simulink model "dstatcom_avg"  (Simulink 7.9)
settings: Solver=ode23tb  SolverMode=SingleTasking  StartTime=0.0  StopTime=12  FixedStep=Ts  MaxStep=1/60  RelTol=1e-4
InitFcn:
  | Ts=40e-6;
  | tic;
StopFcn:
  | toc;
undefined symbols (not defined in the file or in its folder): D11, Delta, DiscIntNeverNeededParam
libraries: powerlib x53, powerlib_extras x39
(part 1 of 2)
Description:
  | Copyright 2008-2012 The MathWorks, Inc.
settings Model: Creator=MathWorks  LastModifiedBy=ywlaw  ExtModeTrigMode=oneshot  ExtModeArmWhenConnect=off  ExtModeAutoUpdateStatusClock=off
settings DataIOCC: LimitDataPoints=off  SaveFinalState=on  SaveFormat=Structure  SaveOutput=off  SaveTime=off  SignalLoggingName=sigsOut
settings OptimizationCC: BlockReduction=off  BooleanDataType=off  InitFltsAndDblsToZero=on
settings DebuggingCC: SaveWithParameterizedLinksMsg=none  SignalResolutionControl=TryResolveAllWithWarning  SolverPrmCheckMsg=none  MultiTaskDSMMsg=warning  MultiTaskCondExecSysMsg=none  FcnCallInpInsideContextMsg=Use local settings  StrictBusMsg=None
settings HardwareCC: TargetUnknown=on
settings RTWCC: IncludeERTFirstTime=on
settings GRTTargetCC: TargetFcnLib=ansi_tfl_tmw.mat  CombineOutputUpdateFcns=off  GRTInterface=on

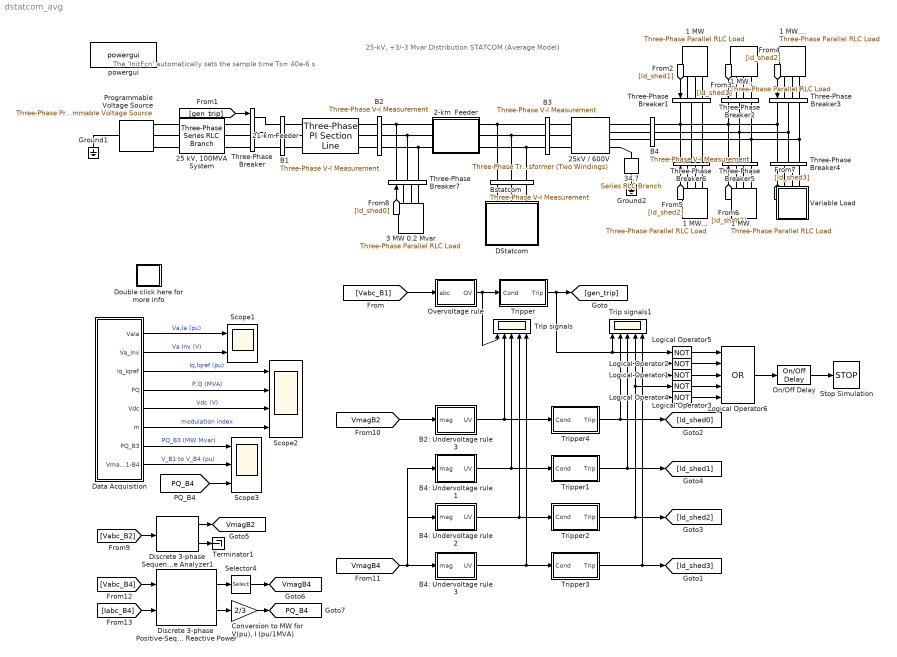
== system dstatcom_avg ==
  note: 25-kV, +3/-3 Mvar Distribution STATCOM (Average Model)
  note: The 'InitFcn' automatically sets
      |  the sample time Ts= 40e-6 s
  1 MW : powerlib/Elements/Three-Phase Parallel RLC Load  LConnTagsString=A|B|C  Configuration=Y (floating)  NominalVoltage=600  NominalFrequency=60  ActivePower=1e6  InductivePower=0  CapacitivePower=0  Measurements=None  LoadType=constant Z
  1 MW. : powerlib/Elements/Three-Phase Parallel RLC Load  LConnTagsString=A|B|C  Configuration=Y (floating)  NominalVoltage=600  NominalFrequency=60  ActivePower=1e6  InductivePower=0  CapacitivePower=0  Measurements=None  LoadType=constant Z
  1 MW.. : powerlib/Elements/Three-Phase Parallel RLC Load  LConnTagsString=A|B|C  Configuration=Y (floating)  NominalVoltage=600  NominalFrequency=60  ActivePower=1e6  InductivePower=0  CapacitivePower=0  Measurements=None  LoadType=constant Z
  1 MW... : powerlib/Elements/Three-Phase Parallel RLC Load  LConnTagsString=A|B|C  Configuration=Y (floating)  NominalVoltage=600  NominalFrequency=60  ActivePower=1e6  InductivePower=0  CapacitivePower=0  Measurements=None  LoadType=constant Z
  1 MW.... : powerlib/Elements/Three-Phase Parallel RLC Load  LConnTagsString=A|B|C  Configuration=Y (floating)  NominalVoltage=600  NominalFrequency=60  ActivePower=1e6  InductivePower=0  CapacitivePower=0  Measurements=None  LoadType=constant Z
  2-km  Feeder : Subsystem
      mask Display: plot(0,0,100,100,[20,20,80,80,90,80,80,20,20,10],[50,40,40,50,50,50,61,61,50,50])
  21-km Feeder : powerlib/Elements/Three-Phase PI Section Line  LConnTagsString=a|b|c  RConnTagsString=A|B|C  Frequency=60  Resistances=[0.1153 0.3963]  Inductances=[1.048e-3 2.730e-3]  Capacitances=[11.33e-9 5.338e-9]  Length=21
  "25 kV, 100MVA System" : powerlib/Elements/Three-Phase Series RLC Branch  LConnTagsString=A|B|C  RConnTagsString=A|B|C  BranchType=RL  Resistance=25e3^2/100e6/10  Inductance=25e3^2/100e6/(2*pi*60)  Capacitance=1.0  Measurements=None
  25kV / 600V : powerlib/Elements/Three-Phase Transformer (Two Windings)  Winding1Connection=Delta (D11)  UNITS=pu  NominalPower=[6e6 60]  Winding1=[25e3 , 0.05/30/2 , 0.05]  Winding2Connection=Yn  Winding2=[600 , 0.05/30/2 , 0]  SetSaturation=off  Rm=500  Lm=500  Saturation="[ 0,0  ;  0.005,1.2  ;  1.0,1.4 ]"  Hysteresis=off  DataFile='basic_model'  SetInitialFlux=off  InitialFluxes=[ 0.8 , -0.8 , 0.7 ]  Measurements=None  MoreParameters=off  BreakLoop=off  DataType=off  TransfoNumber=1
  3 MW 0.2 Mvar : powerlib/Elements/Three-Phase Parallel RLC Load  LConnTagsString=A|B|C  Configuration=Y (grounded)  NominalVoltage=25e3  NominalFrequency=60  ActivePower=3e6  InductivePower=0  CapacitivePower=0.2e6  Measurements=None  LoadType=constant Z
  34.7 : powerlib/Elements/Series RLC Branch  LConnTagsString=__new0  RConnTagsString=__new0  BranchType=R  Resistance=34.7  Inductance=1.0  SetiL0=off  InitialCurrent=0  Capacitance=1.0  Setx0=off  InitialVoltage=0  Measurements=None
  B1 : powerlib/Measurements/Three-Phase V-I Measurement  VoltageMeasurement=phase-to-ground  SetLabelV=on  LabelV=Vabc_B1  Vpu=on  VpuLL=off  CurrentMeasurement=no  SetLabelI=off  LabelI=Iabc  Ipu=off  Pbase=100e6  Vbase=25e3  OutputType=Complex  PhasorSimulation=off  PSBequivalent=0
  B2 : powerlib/Measurements/Three-Phase V-I Measurement  VoltageMeasurement=phase-to-ground  SetLabelV=on  LabelV=Vabc_B2  Vpu=on  VpuLL=off  CurrentMeasurement=no  SetLabelI=off  LabelI=Iabc  Ipu=off  Pbase=100e6  Vbase=25e3  OutputType=Complex  PhasorSimulation=off  PSBequivalent=0
  B2: Undervoltage rule 3 : Subsystem  mask{Freq=60, Vmin=[ 0.94, 6 ]}
      mask prompts: Freq "Fundamental frequency (Hz)"; Vmin "[Minimum voltage (p.u.), Delay (s)]"
      mask init:
      | Min_V1 = Vmin(1);
      | Delay_V1 = Vmin(2);
      | a = exp(2*pi*j/3);
      | a2 = a^2;
  B3 : powerlib/Measurements/Three-Phase V-I Measurement  VoltageMeasurement=phase-to-ground  SetLabelV=on  LabelV=Vabc_B3  Vpu=on  VpuLL=off  CurrentMeasurement=yes  SetLabelI=on  LabelI=Iabc_B3  Ipu=on  Pbase=1e6  Vbase=25e3  OutputType=Magnitude  PhasorSimulation=off  PSBequivalent=0
  B4 : powerlib/Measurements/Three-Phase V-I Measurement  VoltageMeasurement=phase-to-ground  SetLabelV=on  LabelV=Vabc_B4  Vpu=on  VpuLL=off  CurrentMeasurement=yes  SetLabelI=on  LabelI=Iabc_B4  Ipu=on  Pbase=1e6  Vbase=600  OutputType=Magnitude  PhasorSimulation=off  PSBequivalent=0
  B4: Undervoltage rule 1 : Subsystem  mask{Freq=60, Vmin=[ 0.94, 6 ]}
      mask prompts: Freq "Fundamental frequency (Hz)"; Vmin "[Minimum voltage (p.u.), Delay (s)]"
      mask init:
      | Min_V1 = Vmin(1);
      | Delay_V1 = Vmin(2);
      | a = exp(2*pi*j/3);
      | a2 = a^2;
  B4: Undervoltage rule 2 : Subsystem  mask{Freq=60, Vmin=[ 0.92, 3 ]}
      mask prompts: Freq "Fundamental frequency (Hz)"; Vmin "[Minimum voltage (p.u.), Delay (s)]"
      mask init:
      | Min_V1 = Vmin(1);
      | Delay_V1 = Vmin(2);
      | a = exp(2*pi*j/3);
      | a2 = a^2;
  B4: Undervoltage rule 3 : Subsystem  mask{Freq=60, Vmin=[ 0.90, 1.5 ]}
      mask prompts: Freq "Fundamental frequency (Hz)"; Vmin "[Minimum voltage (p.u.), Delay (s)]"
      mask init:
      | Min_V1 = Vmin(1);
      | Delay_V1 = Vmin(2);
      | a = exp(2*pi*j/3);
      | a2 = a^2;
  Bstatcom : powerlib/Measurements/Three-Phase V-I Measurement  VoltageMeasurement=phase-to-ground  SetLabelV=on  LabelV=Vabc_Bstatcom  Vpu=on  VpuLL=off  CurrentMeasurement=yes  SetLabelI=on  LabelI=Iabc_Bstatcom  Ipu=on  Pbase=3e6  Vbase=25e3  OutputType=Magnitude  PhasorSimulation=off  PSBequivalent=0
  "Conversion to MW for V(pu), I (pu/1MVA)" : Gain  Gain=2/3  SaturateOnIntegerOverflow=on  OutDataTypeStr=Inherit: Same as input  ParamDataTypeStr=Inherit: Same as input
  DStatcom : Subsystem
      mask Display: disp('D-STATCOM\n+/- 3Mvar\nAverage')
  Data Acquisition : Subsystem
  Discrete 3-phase Sequence Analyzer1 : powerlib_extras/Discrete Measurements/Discrete 3-phase Sequence Analyzer  Freq=60  n=1  seq=Positive  Par_Init=[1 0]  Ts=Ts
  Discrete 3-phase  Positive-Sequence  Active & Reactive Power : powerlib_extras/Discrete Measurements/Discrete 3-phase  Positive-Sequence  Active & Reactive Power  Freq=60  Par_Vinit=[1 0]  Par_Iinit=[0 0]  Ts=Ts
  Double click here for more info : Subsystem
      settings: OpenFcn=showdemo(bdroot(gcb))
      mask Display: disp('?')
  Ground1 : powerlib/Elements/Ground  LConnTagsString=a
  Ground2 : powerlib/Elements/Ground  LConnTagsString=a
  Logical Operator{1..5} (5 alike) : Logic  Operator=NOT  AllPortsSameDT=off
  Logical Operator6 : Logic  Operator=OR  Inputs=5  AllPortsSameDT=off
  On/Off Delay : powerlib_extras/Control  Blocks/On//Off Delay  type_delay=On delay  delay=0.1  ic=0
  Overvoltage rule : Subsystem  mask{Freq=60, Vmax=[ 1.1, 1.5 ]}
      mask prompts: Freq "Fundamental frequency (Hz)"; Vmax "[Maximum voltage (p.u.), Delay (s)]"
      mask init:
      | Max_V1 = Vmax(1);
      | Delay_V1 = Vmax(2);
      | a = exp(2*pi*j/3);
      | a2 = a^2;
  Programmable Voltage Source : powerlib/Electrical Sources/Three-Phase Programmable Voltage Source  PositiveSequence=[(26925)*1 0 60]  VariationEntity=None  VariationType=Table of time-amplitude pairs  VariationTypeAlt=Step  VariationStep=0.5  VariationRate=10  VariationMagnitude=0.3  VariationFrequency=2  VariationTiming=[1 2]  VariationPhaseA=off  Amplitudes=[1 1.06 0.94 1.0]  TimeValues=[0 0.2 0.3 0.4]  HarmonicGeneration=off  HarmonicA=[3 0.2 -25 0]  HarmonicB=[2 0.15 35 2]  Timing="[0.05  3]"  BusType=swing  Pref=0  Qref=0  Qmin=-inf  Qmax=inf
  Scope1 : Scope  NumInputPorts=2
      settings: TimeRange=0.5  YMin=-1.5~-4000  YMax=1.5~4000  SaveName=Sig1  SampleInput=on  SampleTime=Ts
  Scope2 : Scope  NumInputPorts=4
      settings: ShowLegends=on  TimeRange=1  YMin=-1.5~-4~2200~0.4  YMax=1.5~4~2600~1.2  SaveName=Scope2  SampleInput=on  SampleTime=Ts*32
  Scope3 : Scope  NumInputPorts=3
      settings: ShowLegends=on  TimeRange=1  YMin=0~0.725~-3.5  YMax=6~1~3.5  SaveName=Scope3  SampleInput=on  SampleTime=Ts
  Selector4 : Selector  InputPortWidth=2  IndexOptions=Index vector (dialog)  Indices=1  OutputSizes=1
  Stop Simulation : Stop
  Terminator1 : Terminator
  Three-Phase Breaker{,1..7} (8 alike) : powerlib/Elements/Three-Phase Breaker  InitialState=closed  SwitchA=on  SwitchB=on  SwitchC=on  SwitchTimes="[4/60  10/60]"  External=on  BreakerResistance=0.001  SnubberResistance=1e6  SnubberCapacitance=inf  Measurements=None
  Trip signals : Scope  NumInputPorts=5
      settings: ShowLegends=on  YMin=0~-5~-5~-5~-5  YMax=6~5~5~5~5  SaveName=Sig10  SampleInput=on  SampleTime=Ts
  Trip signals1 : Scope  NumInputPorts=5
      settings: ShowLegends=on  TimeRange=0.5  YMin=0~-5~-5~-5~-5  YMax=6~5~5~5~5  SaveName=Sig11  SampleInput=on  SampleTime=Ts
  Tripper : Subsystem
  Tripper1 : Subsystem
  Tripper2 : Subsystem
  Tripper3 : Subsystem
  Tripper4 : Subsystem
  Variable Load : Subsystem  mask(Variable Load (Constant Current)){Par_Nom=[3000 0.9], Par_Mod=[2000  5], Par_Time=[0.15 20], Vbase=600, Ts=Ts}
      mask prompts: Par_Nom "Nominal load: [ Current (Arms)    Power factor (0 a 1) ]"; Par_Mod "Modulation: [ Amplitude (Arms)   Frequency (Hz) ]"; Par_Time "Modulation timing : [ Ton  Toff ]"; Vbase "Nominal voltage (Volts rms ph-ph)"; Ts "Sample time:"
      mask init:
      | NomAmp=Par_Nom(1)*sqrt(2);
      | NomPha=-acos(Par_Nom(2));
      | ModFreq=Par_Mod(2);
      | ModAmp=Par_Mod(1)*sqrt(2);
      | Ton=Par_Time(1);
      | Toff=Par_Time(2);
  powergui : powerlib/powergui  Priority=2  SimulationMode=Discrete  SolverType=Tustin  SampleTime=Ts  frequency=60  SPID=off  DisableSnubberDevices=off  DisableRonSwitches=off  DisableVfSwitches=off  SwTol=0  Interpol=off  DisplayEquations=off  FunctionMessages=off  frequencyindice=0  Pbase=100e6  ErrMax=1e-4  Iterations=50  UnitsV=kV  UnitsW=MW  echomessages=off  HookPort=off  EnableUseOfTLC=off  x0status=blocks  RestoreLinks=warning  ResistiveCurrentMeasurement=off  Frange=[0:2:500]  Ylog=off  Xlog=on  ShowGrid=off  save=off  variable=ZData  structure=Sig1  ZoomFFT=on  StartTime=0.26  cycles=2  DisplayStyle=1  fundamental=60  FreqAxis=off  MaxFrequency=5000  frequencyindicesteady=1  RmsSteady=1  display=off  Ts=0  methode=off
  tag scope: PQ_B4=global, VmagB2=global, VmagB4=global
  wires:
  Data Acquisition/1(VaIa) -> Scope1/1  "Va,Ia (pu)"
  Data Acquisition/2(Va_Inv) -> Scope1/2  "Va Inv (V)"
  Data Acquisition/5(Vdc) -> Scope2/3  "Vdc (V)"
  Data Acquisition/4(PQ) -> Scope2/2  "P,Q (MVA)"
  Data Acquisition/3(Iq_Iqref) -> Scope2/1  "Iq,Iqref (pu)"
  Data Acquisition/6(m) -> Scope2/4  "modulation index"
  Data Acquisition/7(PQ_B3) -> Scope3/1  "PQ_B3 (MW Mvar)"
  Data Acquisition/8(VmagB1-B4) -> Scope3/2  "V_B1 to V_B4 (pu)"
  [gen_trip] -> Three-Phase Breaker/1
  [ld_shed1] -> Three-Phase Breaker1/1
  [ld_shed1] -> Three-Phase Breaker2/1
  [ld_shed2] -> Three-Phase Breaker3/1
  [ld_shed2] -> Three-Phase Breaker6/1
  [ld_shed3] -> Three-Phase Breaker5/1
  [ld_shed3] -> Three-Phase Breaker4/1
  Overvoltage rule/1(OV) -> Tripper/1(Cond), Trip signals/1
  Tripper/1(Trip) -> [gen_trip], Trip signals1/1, Logical Operator5/1
  Tripper1/1(Trip) -> [ld_shed1], Trip signals1/3, Logical Operator1/1
  Tripper2/1(Trip) -> [ld_shed2], Trip signals1/4, Logical Operator3/1
  Tripper3/1(Trip) -> [ld_shed3], Trip signals1/5, Logical Operator4/1
  [Vabc_B1] -> Overvoltage rule/1(abc)
  [VmagB4] -> B4: Undervoltage rule 1/1(mag), B4: Undervoltage rule 2/1(mag), B4: Undervoltage rule 3/1(mag)
  B4: Undervoltage rule 1/1(UV) -> Tripper1/1(Cond), Trip signals/3
  B4: Undervoltage rule 2/1(UV) -> Tripper2/1(Cond), Trip signals/4
  B4: Undervoltage rule 3/1(UV) -> Tripper3/1(Cond), Trip signals/5
  [ld_shed0] -> Three-Phase Breaker7/1
  Tripper4/1(Trip) -> [ld_shed0], Trip signals1/2, Logical Operator2/1
  B2: Undervoltage rule 3/1(UV) -> Tripper4/1(Cond), Trip signals/2
  [Vabc_B2] -> Discrete 3-phase Sequence Analyzer1/1
  Discrete 3-phase Sequence Analyzer1/2 -> Terminator1/1
  Discrete 3-phase Sequence Analyzer1/1 -> [VmagB2]
  [VmagB2] -> B2: Undervoltage rule 3/1(mag)
  [Vabc_B4] -> Discrete 3-phase  Positive-Sequence  Active & Reactive Power/1
  [Iabc_B4] -> Discrete 3-phase  Positive-Sequence  Active & Reactive Power/2
  Discrete 3-phase  Positive-Sequence  Active & Reactive Power/2 -> "Conversion to MW for V(pu), I (pu/1MVA)"/1
  Discrete 3-phase  Positive-Sequence  Active & Reactive Power/1 -> Selector4/1
  Selector4/1 -> [VmagB4]
  "Conversion to MW for V(pu), I (pu/1MVA)"/1 -> [PQ_B4]
  [PQ_B4] -> Scope3/3
  Logical Operator5/1 -> Logical Operator6/1
  Logical Operator2/1 -> Logical Operator6/2
  Logical Operator1/1 -> Logical Operator6/3
  Logical Operator3/1 -> Logical Operator6/4
  Logical Operator4/1 -> Logical Operator6/5
  Logical Operator6/1 -> On/Off Delay/1
  On/Off Delay/1 -> Stop Simulation/1
  connections:
  B3/LConn2 -- 2-km  Feeder/RConn2 -- Bstatcom/LConn2
  2-km  Feeder/RConn1 -- B3/LConn1 -- Bstatcom/LConn1
  B3/LConn3 -- 2-km  Feeder/RConn3 -- Bstatcom/LConn3
  34.7/RConn1 -- Ground2/LConn1
  25kV / 600V/RConn4 -- 34.7/LConn1
  Programmable Voltage Source/RConn1 -- "25 kV, 100MVA System"/LConn1
  Programmable Voltage Source/RConn2 -- "25 kV, 100MVA System"/LConn2
  Programmable Voltage Source/RConn3 -- "25 kV, 100MVA System"/LConn3
  Ground1/LConn1 -- Programmable Voltage Source/LConn1
  21-km Feeder/RConn1 -- B2/LConn1
  21-km Feeder/RConn2 -- B2/LConn2
  21-km Feeder/RConn3 -- B2/LConn3
  2-km  Feeder/LConn1 -- B2/RConn1 -- Three-Phase Breaker7/RConn1
  2-km  Feeder/LConn2 -- B2/RConn2 -- Three-Phase Breaker7/RConn2
  Bstatcom/RConn3 -- DStatcom/RConn3
  DStatcom/RConn1 -- Bstatcom/RConn1
  DStatcom/RConn2 -- Bstatcom/RConn2
  B3/RConn1 -- 25kV / 600V/LConn1
  B3/RConn2 -- 25kV / 600V/LConn2
  B3/RConn3 -- 25kV / 600V/LConn3
  25kV / 600V/RConn1 -- B4/RConn1
  25kV / 600V/RConn2 -- B4/RConn2
  25kV / 600V/RConn3 -- B4/RConn3
  Three-Phase Breaker3/RConn1 -- Three-Phase Breaker2/RConn1 -- Three-Phase Breaker1/RConn1 -- B4/LConn1 -- Three-Phase Breaker6/RConn1 -- Three-Phase Breaker5/RConn1 -- Three-Phase Breaker4/RConn1
  Three-Phase Breaker2/RConn3 -- B4/LConn3 -- Three-Phase Breaker1/RConn3 -- Three-Phase Breaker6/RConn3 -- Three-Phase Breaker5/RConn3 -- Three-Phase Breaker3/RConn3 -- Three-Phase Breaker4/RConn3
  "25 kV, 100MVA System"/RConn1 -- Three-Phase Breaker/LConn1
  "25 kV, 100MVA System"/RConn2 -- Three-Phase Breaker/LConn2
  "25 kV, 100MVA System"/RConn3 -- Three-Phase Breaker/LConn3
  Three-Phase Breaker/RConn2 -- B1/LConn2
  Three-Phase Breaker/RConn3 -- B1/LConn3
  Three-Phase Breaker/RConn1 -- B1/LConn1
  2-km  Feeder/LConn3 -- B2/RConn3 -- Three-Phase Breaker7/RConn3
  B1/RConn1 -- 21-km Feeder/LConn1
  B1/RConn2 -- 21-km Feeder/LConn2
  B1/RConn3 -- 21-km Feeder/LConn3
  Three-Phase Breaker1/LConn3 -- 1 MW/LConn3
  Three-Phase Breaker1/LConn2 -- 1 MW/LConn2
  Three-Phase Breaker1/LConn1 -- 1 MW/LConn1
  Three-Phase Breaker2/LConn3 -- 1 MW../LConn3
  Three-Phase Breaker2/LConn2 -- 1 MW../LConn2
  Three-Phase Breaker2/LConn1 -- 1 MW../LConn1
  1 MW..../LConn1 -- Three-Phase Breaker3/LConn1
  1 MW..../LConn2 -- Three-Phase Breaker3/LConn2
  1 MW..../LConn3 -- Three-Phase Breaker3/LConn3
  Variable Load/LConn1 -- Three-Phase Breaker4/LConn1
  Variable Load/LConn2 -- Three-Phase Breaker4/LConn2
  Variable Load/LConn3 -- Three-Phase Breaker4/LConn3
  1 MW./LConn1 -- Three-Phase Breaker5/LConn1
  1 MW./LConn2 -- Three-Phase Breaker5/LConn2
  1 MW./LConn3 -- Three-Phase Breaker5/LConn3
  Three-Phase Breaker2/RConn2 -- B4/LConn2 -- Three-Phase Breaker1/RConn2 -- Three-Phase Breaker6/RConn2 -- Three-Phase Breaker5/RConn2 -- Three-Phase Breaker3/RConn2 -- Three-Phase Breaker4/RConn2
  1 MW.../LConn1 -- Three-Phase Breaker6/LConn1
  1 MW.../LConn2 -- Three-Phase Breaker6/LConn2
  1 MW.../LConn3 -- Three-Phase Breaker6/LConn3
  Three-Phase Breaker7/LConn1 -- 3 MW 0.2 Mvar/LConn1
  Three-Phase Breaker7/LConn2 -- 3 MW 0.2 Mvar/LConn2
  Three-Phase Breaker7/LConn3 -- 3 MW 0.2 Mvar/LConn3

== system dstatcom_avg/2-km  Feeder ==
  Three-Phase Mutual Inductance Z1-Z0 : powerlib/Elements/Three-Phase Mutual Inductance Z1-Z0  LConnTagsString=a|b|c  RConnTagsString=A|B|C  PositiveSequence="[0.1153  1.048e-3]*2"  ZeroSequence="[0.3963  2.730e-3]*2"
  A : PMIOPort  Port=1  Side=Left
  B : PMIOPort  Port=2  Side=Left
  "C " : PMIOPort  Port=3  Side=Left
  a : PMIOPort  Port=4  Side=Right
  b : PMIOPort  Port=5  Side=Right
  c : PMIOPort  Port=6  Side=Right
  connections:
  Three-Phase Mutual Inductance Z1-Z0/RConn3 -- c/RConn1
  Three-Phase Mutual Inductance Z1-Z0/RConn2 -- b/RConn1
  Three-Phase Mutual Inductance Z1-Z0/RConn1 -- a/RConn1
  "C "/RConn1 -- Three-Phase Mutual Inductance Z1-Z0/LConn3
  B/RConn1 -- Three-Phase Mutual Inductance Z1-Z0/LConn2
  A/RConn1 -- Three-Phase Mutual Inductance Z1-Z0/LConn1

== system dstatcom_avg/B2: Undervoltage rule 3 ==
  mag : Inport
  On/Off Delay : powerlib_extras/Control  Blocks/On//Off Delay  type_delay=On delay  delay=Delay_V1  ic=0
  Relational Operator : RelationalOperator  Operator=<  OutDataTypeStr=boolean
  V0/V1 max1 : Constant  Value=Min_V1
  UV : Outport
  wires:
  V0/V1 max1/1 -> Relational Operator/2
  mag/1 -> Relational Operator/1
  Relational Operator/1 -> On/Off Delay/1
  On/Off Delay/1 -> UV/1

== system dstatcom_avg/B4: Undervoltage rule 1 ==
  mag : Inport
  On/Off Delay : powerlib_extras/Control  Blocks/On//Off Delay  type_delay=On delay  delay=Delay_V1  ic=0
  Relational Operator : RelationalOperator  Operator=<  OutDataTypeStr=boolean
  V0/V1 max1 : Constant  Value=Min_V1
  UV : Outport
  wires:
  V0/V1 max1/1 -> Relational Operator/2
  mag/1 -> Relational Operator/1
  Relational Operator/1 -> On/Off Delay/1
  On/Off Delay/1 -> UV/1

== system dstatcom_avg/B4: Undervoltage rule 2 ==
  mag : Inport
  On/Off Delay2 : powerlib_extras/Control  Blocks/On//Off Delay  type_delay=On delay  delay=Delay_V1  ic=0
  Relational Operator7 : RelationalOperator  Operator=<
  V0/V1 max5 : Constant  Value=Min_V1
  UV : Outport
  wires:
  On/Off Delay2/1 -> UV/1
  V0/V1 max5/1 -> Relational Operator7/2
  mag/1 -> Relational Operator7/1
  Relational Operator7/1 -> On/Off Delay2/1

== system dstatcom_avg/B4: Undervoltage rule 3 ==
  mag : Inport
  On/Off Delay2 : powerlib_extras/Control  Blocks/On//Off Delay  type_delay=On delay  delay=Delay_V1  ic=0
  Relational Operator7 : RelationalOperator  Operator=<
  V0/V1 max5 : Constant  Value=Min_V1
  UV : Outport
  wires:
  On/Off Delay2/1 -> UV/1
  V0/V1 max5/1 -> Relational Operator7/2
  Relational Operator7/1 -> On/Off Delay2/1
  mag/1 -> Relational Operator7/1

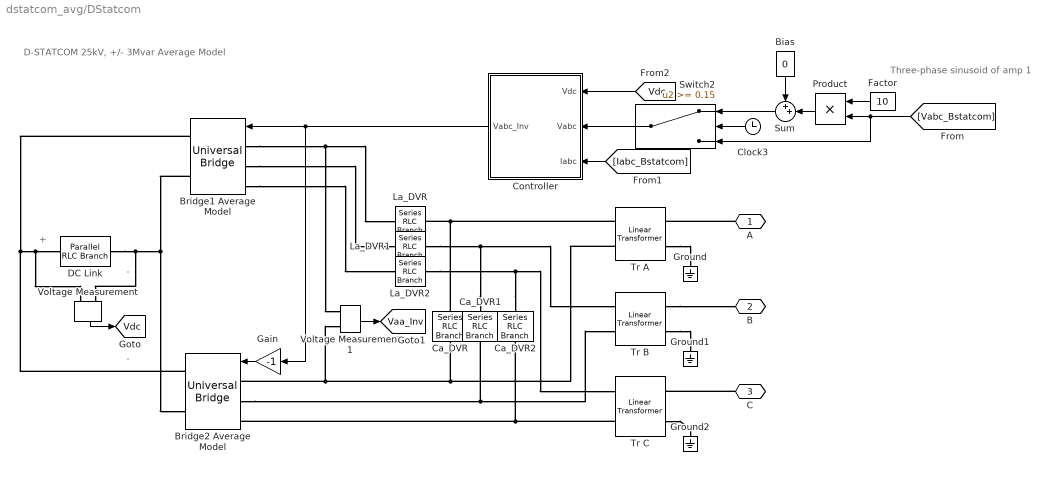
== system dstatcom_avg/DStatcom ==
  note: D-STATCOM
      | 25kV, +/- 3Mvar
      | Average Model
  note: +
  note: -
  note: -
  note: Three-phase sinusoid
      | of amp 1
  Bias : Constant  Value=0
  Bridge1 Average Model : powerlib/Power Electronics/Universal Bridge  Arms=3  SnubberResistance=1e5  SnubberCapacitance=inf  Device=Average-model based VSC  Ron=1e-3  Lon=0  ForwardVoltages="[  0  0  ]"  ForwardVoltage=0  GTOparameters=[ 10e-6 , 20e-6 ]  IGBTparameters=[ 1e-6 , 2e-6 ]  Measurements=None  Measurements_2=None  converterType=Rectifier
  Bridge2 Average Model : powerlib/Power Electronics/Universal Bridge  Arms=3  SnubberResistance=1e5  SnubberCapacitance=inf  Device=Average-model based VSC  Ron=1e-3  Lon=0  ForwardVoltages="[  0  0  ]"  ForwardVoltage=0  GTOparameters=[ 10e-6 , 20e-6 ]  IGBTparameters=[ 1e-6 , 2e-6 ]  Measurements=None  Measurements_2=None  converterType=Rectifier
  Ca_DVR : powerlib/Elements/Series RLC Branch  LConnTagsString=__new0  RConnTagsString=__new0  BranchType=RC  Resistance=100e-6*(2*pi*60)/40  Inductance=1.0  SetiL0=off  InitialCurrent=0  Capacitance=100e-6  Setx0=off  InitialVoltage=0  Measurements=None
  Ca_DVR1 : powerlib/Elements/Series RLC Branch  LConnTagsString=__new0  RConnTagsString=__new0  BranchType=RC  Resistance=100e-6*(2*pi*60)/40  Inductance=1.0  SetiL0=off  InitialCurrent=0  Capacitance=100e-6  Setx0=off  InitialVoltage=0  Measurements=None
  Ca_DVR2 : powerlib/Elements/Series RLC Branch  LConnTagsString=__new0  RConnTagsString=__new0  BranchType=RC  Resistance=100e-6*(2*pi*60)/40  Inductance=1.0  SetiL0=off  InitialCurrent=0  Capacitance=100e-6  Setx0=off  InitialVoltage=0  Measurements=None
  Clock3 : Clock
  Controller : Subsystem  mask(D-STATCOM Controller){ModeOper=Voltage regulation, Vac_Ref=1.0, Qref=0, Vdc_Ref=2400, Par_VacReg=[0.55 2500], Par_VdcReg=[0.001 0.15], Par_IReg=[0.8 200 0], Ts=Ts}
      mask prompts: ModeOper "Mode of operation:"; Vac_Ref "AC voltage setpoint Vref (pu):"; Qref "Manual mode: Qref (Reactive power in pu):"; Vdc_Ref "DC Voltage setpoint (Volts)"; Par_VacReg "Vac Regulator Gains: [ Kp  Ki ]"; Par_VdcReg "Vdc Regulator Gains: [ Kp  Ki ]"; Par_IReg "Current Regulators Gain: [ Kp Ki Kd ]"; Ts "Sample time (s)"
      mask init:
      | Kp_I=Par_IReg(1);
      | Ki_I=Par_IReg(2);
      | Kd_I=Par_IReg(3);
      | Kp_Vdc=Par_VdcReg(1);
      | Ki_Vdc=Par_VdcReg(2);
      | Kp_Vac=Par_VacReg(1);
      | Ki_Vac=Par_VacReg(2);
      mask StyleString: popup(Voltage regulation|Q regulation),edit,edit,edit,edit,edit,edit,edit
  DC Link : powerlib/Elements/Parallel RLC Branch  LConnTagsString=a  RConnTagsString=__new0  BranchType=C  Resistance=1.0  Inductance=1.0  SetiL0=off  InitialCurrent=0  Capacitance=10000e-6  Setx0=off  InitialVoltage=0  Measurements=None
  Factor : Constant  Value=10
  Gain : Gain  Gain=-1
  Ground : powerlib/Elements/Ground  LConnTagsString=a
  Ground1 : powerlib/Elements/Ground  LConnTagsString=a
  Ground2 : powerlib/Elements/Ground  LConnTagsString=a
  La_DVR : powerlib/Elements/Series RLC Branch  LConnTagsString=__new0  RConnTagsString=__new0  BranchType=L  Resistance=1.0  Inductance=800e-6  SetiL0=off  InitialCurrent=0  Capacitance=1.0  Setx0=off  InitialVoltage=0  Measurements=None
  La_DVR1 : powerlib/Elements/Series RLC Branch  LConnTagsString=__new0  RConnTagsString=__new0  BranchType=L  Resistance=1.0  Inductance=800e-6  SetiL0=off  InitialCurrent=0  Capacitance=1.0  Setx0=off  InitialVoltage=0  Measurements=None
  La_DVR2 : powerlib/Elements/Series RLC Branch  LConnTagsString=__new0  RConnTagsString=__new0  BranchType=L  Resistance=1.0  Inductance=800e-6  SetiL0=off  InitialCurrent=0  Capacitance=1.0  Setx0=off  InitialVoltage=0  Measurements=None
  Product : Product  RndMeth=Zero
  Sum : Sum  Inputs=++|
  Switch2 : Switch  Threshold=0.15
  Tr A : powerlib/Elements/Linear Transformer  LConnTagsString=a|b  RConnTagsString=A|B  UNITS=pu  NominalPower=[3e6/3 60]  winding1=[1250 0.03/30 0.03]  winding2=[25e3/sqrt(3) 0.03/30 0.03]  ThreeWindings=off  winding3=[60e3 0.005 0.02]  RmLm=[200 200]  Measurements=None  DataType=off
  Tr B : powerlib/Elements/Linear Transformer  LConnTagsString=a|b  RConnTagsString=A|B  UNITS=pu  NominalPower=[3e6/3 60]  winding1=[1250 0.03/30 0.03]  winding2=[25e3/sqrt(3) 0.03/30 0.03]  ThreeWindings=off  winding3=[60e3 0.005 0.02]  RmLm=[200 200]  Measurements=None  DataType=off
  Tr C : powerlib/Elements/Linear Transformer  LConnTagsString=a|b  RConnTagsString=A|B  UNITS=pu  NominalPower=[3e6/3 60]  winding1=[1250 0.03/30 0.03]  winding2=[25e3/sqrt(3) 0.03/30 0.03]  ThreeWindings=off  winding3=[60e3 0.005 0.02]  RmLm=[200 200]  Measurements=None  DataType=off
  Voltage Measurement : powerlib/Measurements/Voltage Measurement  Tag=PoWeRsYsTeMmEaSuReMeNt  PhasorSimulation=off  OutputType=Magnitude  PSBequivalent=0
  Voltage Measurement1 : powerlib/Measurements/Voltage Measurement  Tag=PoWeRsYsTeMmEaSuReMeNt  PhasorSimulation=off  OutputType=Magnitude  PSBequivalent=0
  A : PMIOPort  Port=1  Side=Right
  B : PMIOPort  Port=2  Side=Right
  C : PMIOPort  Port=3  Side=Right
  tag scope: Vaa_Inv=global, Vdc=global
  wires:
  [Iabc_Bstatcom] -> Controller/3(Iabc)
  Voltage Measurement/1 -> [Vdc]
  [Vdc] -> Controller/1(Vdc)
  Controller/1(Vabc_Inv) -> Bridge1 Average Model/1, Gain/1
  Gain/1 -> Bridge2 Average Model/1
  Voltage Measurement1/1 -> [Vaa_Inv]
  [Vabc_Bstatcom] -> Product/2, Switch2/3
  Factor/1 -> Product/1
  Product/1 -> Sum/2
  Bias/1 -> Sum/1
  Switch2/1 -> Controller/2(Vabc)
  Clock3/1 -> Switch2/2
  Sum/1 -> Switch2/1
  connections:
  Bridge2 Average Model/LConn2 -- Ca_DVR1/LConn1 -- Tr B/LConn2
  Tr C/LConn2 -- Ca_DVR2/LConn1 -- Bridge2 Average Model/LConn3
  Ca_DVR1/RConn1 -- La_DVR1/RConn1 -- Tr B/LConn1
  Ca_DVR2/RConn1 -- La_DVR2/RConn1 -- Tr C/LConn1
  Tr A/LConn1 -- La_DVR/RConn1 -- Ca_DVR/RConn1
  Tr C/RConn2 -- Ground2/LConn1
  Tr B/RConn2 -- Ground1/LConn1
  Tr A/RConn2 -- Ground/LConn1
  A/RConn1 -- Tr A/RConn1
  Tr B/RConn1 -- B/RConn1
  C/RConn1 -- Tr C/RConn1
  Tr A/LConn2 -- Ca_DVR/LConn1 -- Bridge2 Average Model/LConn1 -- Voltage Measurement1/LConn2
  Bridge1 Average Model/RConn1 -- Bridge2 Average Model/RConn1 -- DC Link/LConn1 -- Voltage Measurement/LConn1
  Bridge1 Average Model/LConn1 -- La_DVR/LConn1 -- Voltage Measurement1/LConn1
  Bridge1 Average Model/LConn2 -- La_DVR1/LConn1
  Bridge1 Average Model/LConn3 -- La_DVR2/LConn1
  DC Link/RConn1 -- Bridge1 Average Model/RConn2 -- Bridge2 Average Model/RConn2 -- Voltage Measurement/LConn2

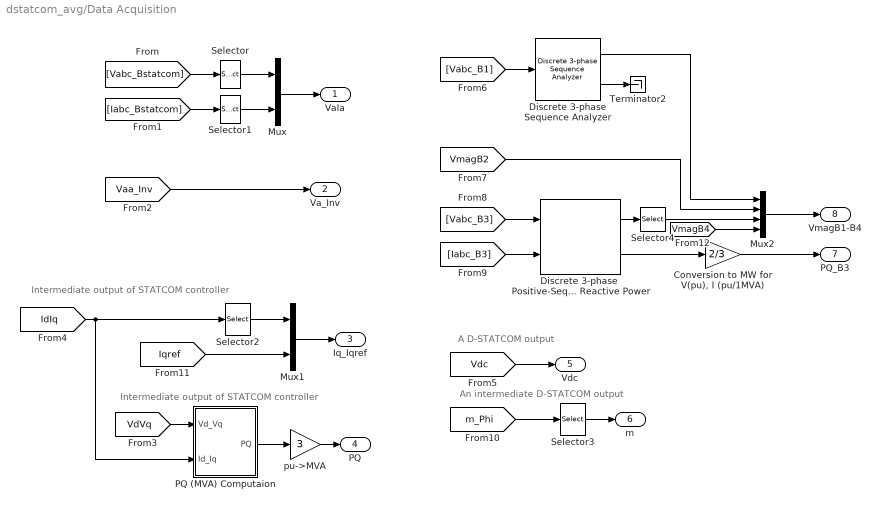
== system dstatcom_avg/Data Acquisition ==
  note: A D-STATCOM output
  note: An intermediate D-STATCOM output
  note: Intermediate output of STATCOM controller
  note: Intermediate output of STATCOM controller
  "Conversion to MW for V(pu), I (pu/1MVA)" : Gain  Gain=2/3  SaturateOnIntegerOverflow=on  OutDataTypeStr=Inherit: Same as input  ParamDataTypeStr=Inherit: Same as input
  Discrete 3-phase Sequence Analyzer : powerlib_extras/Discrete Measurements/Discrete 3-phase Sequence Analyzer  Freq=60  n=1  seq=Positive  Par_Init=[1 0]  Ts=Ts
  Discrete 3-phase  Positive-Sequence  Active & Reactive Power : powerlib_extras/Discrete Measurements/Discrete 3-phase  Positive-Sequence  Active & Reactive Power  Freq=60  Par_Vinit=[1 0]  Par_Iinit=[0 0]  Ts=Ts
  Mux : Mux  Inputs=2
  Mux1 : Mux  Inputs=2
  Mux2 : Mux
  PQ (MVA) Computaion : Subsystem
  Selector : Selector  InputPortWidth=3  IndexOptions=Index vector (dialog)  Indices=1  OutputSizes=1
  Selector1 : Selector  InputPortWidth=3  IndexOptions=Index vector (dialog)  Indices=1  OutputSizes=1
  Selector2 : Selector  InputPortWidth=2  IndexOptions=Index vector (dialog)  Indices=2  OutputSizes=1
  Selector3 : Selector  InputPortWidth=2  IndexOptions=Index vector (dialog)  Indices=1  OutputSizes=1
  Selector4 : Selector  InputPortWidth=2  IndexOptions=Index vector (dialog)  Indices=1  OutputSizes=1
  Terminator2 : Terminator
  pu->MVA : Gain  Gain=3  SaturateOnIntegerOverflow=on  OutDataTypeStr=Inherit: Same as input  ParamDataTypeStr=Inherit: Same as input
  VaIa : Outport
  Va_Inv : Outport  Port=2
  Iq_Iqref : Outport  Port=3
  PQ : Outport  Port=4
  Vdc : Outport  Port=5
  m : Outport  Port=6
  PQ_B3 : Outport  Port=7
  VmagB1-B4 : Outport  Port=8
  wires:
  [Vdc] -> Vdc/1
  [IdIq] -> Selector2/1, PQ (MVA) Computaion/2(Id_Iq)
  Selector/1 -> Mux/1
  Selector1/1 -> Mux/2
  Mux/1 -> VaIa/1
  [m_Phi] -> Selector3/1
  [Vabc_Bstatcom] -> Selector/1
  [Iabc_Bstatcom] -> Selector1/1
  Mux1/1 -> Iq_Iqref/1
  Selector2/1 -> Mux1/1
  [Iqref] -> Mux1/2
  PQ (MVA) Computaion/1(PQ) -> pu->MVA/1
  pu->MVA/1 -> PQ/1
  [VdVq] -> PQ (MVA) Computaion/1(Vd_Vq)
  Selector3/1 -> m/1
  [Vaa_Inv] -> Va_Inv/1
  [Vabc_B3] -> Discrete 3-phase  Positive-Sequence  Active & Reactive Power/1
  [Iabc_B3] -> Discrete 3-phase  Positive-Sequence  Active & Reactive Power/2
  Discrete 3-phase  Positive-Sequence  Active & Reactive Power/2 -> "Conversion to MW for V(pu), I (pu/1MVA)"/1
  [Vabc_B1] -> Discrete 3-phase Sequence Analyzer/1
  Discrete 3-phase Sequence Analyzer/1 -> Mux2/1
  Mux2/1 -> VmagB1-B4/1
  "Conversion to MW for V(pu), I (pu/1MVA)"/1 -> PQ_B3/1
  Discrete 3-phase  Positive-Sequence  Active & Reactive Power/1 -> Selector4/1
  Discrete 3-phase Sequence Analyzer/2 -> Terminator2/1
  Selector4/1 -> Mux2/3
  [VmagB2] -> Mux2/2
  [VmagB4] -> Mux2/4

== system dstatcom_avg/Double click here for more info ==
  note: Run the simulation and observe the following  waveforms on the Scope block:
      |
      | Voltages generated by the inverter (trace 1), load currents (trace 2), phase-neutral voltage and phase-phase voltage of one of  the four inverters (1Y) superimposed on trace 3.
      | When the inverter is operating at no load, you can observe the three 48-step voltage waveform. When the load is switched on the voltage becomes smoother because harmonics
      | are filtered by the transformer leakage reactances.
      |
      | Once the  simulation is completed, open the Powergui and select  "FFT Analysis" to display the 0-4000 Hz frequency spectrum of signals saved
      | in the two "psb48pulse_str" structure. Select signal labeled 'Vabc (pu)'. The FFT will be performed on a 1-cycle window of phase A voltage starting at t = 0.025-1/60 s
      | (inverter operating at no load). Click on Display and observe the frequency spectrum.
      |
      | The fundamental component of  Voltage (in pu) as well as THD  are displayed above the spectrum window.
      | Notice that the first significant harmonics are 47th and 49th (approx. 2%). Notice also that 23rd and 25th are reduced below 0.3%.
      | In order to appreciate the efficiency of harmonic neutralization, you can also observe the frequency spectrum of phase-phase voltage generated by each individual inverter.
      | Select input labeled  "Van Vab Converter 1Y" and signal number 2 and click on Display. Observe that THD in the 0 - 4000 Hz frequency range is 25%.
      |
      | You can also run another simulation by specifying different values of sigma at the input of the pulse generator.
      | You can verify that, in order to cancel a particular harmonic n in the phase-phase voltage of each individual converter, the Sigma value (in degrees) is given by:
      |
      |      Sigma=180*(1 - 1/n)
      |
      | Verify also that choosing Sigma = 180 degrees is equivalent to using 2-level converters and that voltage waveform is degraded to 24 pulses.
  note: In this example, ideal switches and zig-zag phase shifting  transformers are used to build a GTO-type 100 MVA, 138 kV voltage source inverter.
      | This type of converter is used in high-power (up to 200 MVA) Flexible AC Transmission Systems (FACTS) which are used to control power flow on transmission grids.
      | It can be used, for example, to build a model of shunt or series static compensator (STATCOM or SSSC) or, using two such converters, a combination of shunt and series
      | devices known as Unified Power Flow Controller (UPFC).
      |
      | The inverter described in this example is a harmonic neutralized, 48-pulse GTO converter described in reference. It consists of four 3-phase, 3-level inverters and
      | four phase-shifting transformers. Open the "48-pulse inverter" subsystem. Notice that the DC bus (Vdc = +/-9650 V) is connected to the four 3-phase inverters.The four voltages
      | generated by the inverters are applied to secondary windings of four zig-zag phase-shifting transformers connected in Wye (Y) or Delta (D). The four transformer primary windings are
      | connected in series and the converter pulse patterns are phase shifted so that the four voltage fundamental components sum in phase on the primary side.
      |
      | Each 3-level inverter generates three square-wave voltages which can be +Vdc, 0, -Vdc. The duration of the +Vdc or -Vdc level (Sigma) can be adjusted  between 0 and 180
      | degrees from the Sigma input of the Firing Pulse Generator block.
      | Each inverter uses a Three-Level Bridge block where specified power electronic devices are Ideal Switches. In this model each leg of the inverter uses 3 ideal switches
      | to obtain the 3 voltage levels (+Vdc, 0, - Vdc).  This simple model simulates the behavior of a physical inverter where each leg consists of 4 GTOs, 4 antiparallel diodes and
      | 2 neutral clamping diodes. Despite this simplified switch arrangement, the model still requires 4 pulses per arm as in the physical model.
      | The pulse pattern sent to each leg of a 3-phase inverter is described inside the Firing Pulse Generator.
      |
      | You can also select GTO/Diodes pairs instead of Ideal Switches as power electronic devices. It would allow you to specify forward voltage drops for GTOs and diodes
      | and to observe currents flowing in GTOs and diodes  by means of the Multimeter block.
      |
      | The phase shifts produced by the secondary delta connections (-30 degrees) and by the primary zig-zag connections (+7.5 degrees for transformers 1Y and 1D, and -7.5 degrees
      | for transformers 2Y and 2D) allows to neutralize harmonics up to 45th harmonic, as explained below:
      |
      | The 30-degree phase-shift between the Y and D secondaries cancels harmonics 5+12n (5, 17, 29, 41, ...) and 7+12n (7, 19, 31, 43, ...). In addition, the 15-degree phase shift between
      | the two groups of transformers (1Y and 1D leading by 7.5 degrees, 2Y and 2D lagging by +7.5 degrees) allows cancellation of harmonics 11+24n (11, 35, ...) and 13+24n (13, 37, ...).
      | Considering that all 3n the harmonics are not transmitted by the Y and D secondaries, the first harmonic which are not cancelled by the transformers are 23rd, 25th, 47th and 49th.
      | By choosing an appropriate conduction angle for the 3-level inverters (sigma = 180 - 7.5 = 172.5 degrees), the 23rd and 25th can be minimized. The first significant harmonics are
      | therefore the 47th and 49th. This type of inverter generates an almost sinusoidal waveform consisting of  48-steps.
      |
      | The inverter is operated in open loop at constant DC voltage. During the first three cycles the inverter operates at no load. Then, at t = 0.05 s, a 100 MVA resistive load
      | is connected at the 138-kV terminals.
  note: This demonstration illustrates use of 3-level converters and zig-zag phase-shifting
      | transformers in a 48-pulse square-wave GTO converter.  It also demonstrates harmonic
      | analysis using the Powergui/FFT tool.
  note: Circuit Description
  note: Demonstration
  note: P. Giroux and G. Sybille (Hydro-Quebec)
  note: Reference:
  note: Narain G. Hingorani and Laszlo Gyuyi, "Understanding FACTS", IEEE Press , 2000

== system dstatcom_avg/Overvoltage rule ==
  abc : Inport  PortDimensions=3
  Discrete 3-phase Sequence Analyzer : powerlib_extras/Discrete Measurements/Discrete 3-phase Sequence Analyzer  Freq=60  n=1  seq=Positive  Par_Init=[1 0]  Ts=Ts
  On/Off Delay2 : powerlib_extras/Control  Blocks/On//Off Delay  type_delay=On delay  delay=Delay_V1  ic=0
  Relational Operator7 : RelationalOperator  Operator=>
  Terminator3 : Terminator
  V0/V1 max5 : Constant  Value=Max_V1
  OV : Outport
  wires:
  abc/1 -> Discrete 3-phase Sequence Analyzer/1
  On/Off Delay2/1 -> OV/1
  Discrete 3-phase Sequence Analyzer/2 -> Terminator3/1
  Discrete 3-phase Sequence Analyzer/1 -> Relational Operator7/1
  V0/V1 max5/1 -> Relational Operator7/2
  Relational Operator7/1 -> On/Off Delay2/1

== system dstatcom_avg/Tripper ==
  Cond : Inport
  Clock2 : Clock
  Clock3 : Clock
  Constant2 : Constant  Value=0
  Constant3 : Constant
  Logical Operator2 : Logic  Operator=NOT  AllPortsSameDT=off
  Monostable1 : powerlib_extras/Control  Blocks/Monostable  EdgeDetect=Rising  t_mono=1000000  ic=0
  Switch2 : Switch  Threshold=0.15
  Switch3 : Switch  Threshold=0.15
  Trip : Outport
  wires:
  Clock2/1 -> Switch2/2
  Constant2/1 -> Switch2/3
  Constant3/1 -> Switch3/3
  Clock3/1 -> Switch3/2
  Switch2/1 -> Monostable1/1
  Monostable1/1 -> Logical Operator2/1
  Logical Operator2/1 -> Switch3/1
  Cond/1 -> Switch2/1
  Switch3/1 -> Trip/1

== system dstatcom_avg/Tripper1 ==
  Cond : Inport
  Clock2 : Clock
  Clock3 : Clock
  Constant2 : Constant  Value=0
  Constant3 : Constant
  Logical Operator2 : Logic  Operator=NOT  AllPortsSameDT=off
  Monostable1 : powerlib_extras/Control  Blocks/Monostable  EdgeDetect=Rising  t_mono=1000000  ic=0
  Switch2 : Switch  Threshold=0.15
  Switch3 : Switch  Threshold=0.15
  Trip : Outport
  wires:
  Clock2/1 -> Switch2/2
  Constant2/1 -> Switch2/3
  Constant3/1 -> Switch3/3
  Clock3/1 -> Switch3/2
  Switch2/1 -> Monostable1/1
  Monostable1/1 -> Logical Operator2/1
  Logical Operator2/1 -> Switch3/1
  Cond/1 -> Switch2/1
  Switch3/1 -> Trip/1

== system dstatcom_avg/Tripper2 ==
  Cond : Inport
  Clock2 : Clock
  Clock3 : Clock
  Constant2 : Constant  Value=0
  Constant3 : Constant
  Logical Operator2 : Logic  Operator=NOT  AllPortsSameDT=off
  Monostable1 : powerlib_extras/Control  Blocks/Monostable  EdgeDetect=Rising  t_mono=1000000  ic=0
  Switch2 : Switch  Threshold=0.15
  Switch3 : Switch  Threshold=0.15
  Trip : Outport
  wires:
  Clock2/1 -> Switch2/2
  Constant2/1 -> Switch2/3
  Constant3/1 -> Switch3/3
  Clock3/1 -> Switch3/2
  Switch2/1 -> Monostable1/1
  Monostable1/1 -> Logical Operator2/1
  Logical Operator2/1 -> Switch3/1
  Cond/1 -> Switch2/1
  Switch3/1 -> Trip/1

== system dstatcom_avg/Tripper3 ==
  Cond : Inport
  Clock2 : Clock
  Clock3 : Clock
  Constant2 : Constant  Value=0
  Constant3 : Constant
  Logical Operator2 : Logic  Operator=NOT  AllPortsSameDT=off
  Monostable1 : powerlib_extras/Control  Blocks/Monostable  EdgeDetect=Rising  t_mono=1000000  ic=0
  Switch2 : Switch  Threshold=0.15
  Switch3 : Switch  Threshold=0.15
  Trip : Outport
  wires:
  Clock2/1 -> Switch2/2
  Constant2/1 -> Switch2/3
  Constant3/1 -> Switch3/3
  Clock3/1 -> Switch3/2
  Switch2/1 -> Monostable1/1
  Monostable1/1 -> Logical Operator2/1
  Logical Operator2/1 -> Switch3/1
  Cond/1 -> Switch2/1
  Switch3/1 -> Trip/1

== system dstatcom_avg/Tripper4 ==
  Cond : Inport
  Clock2 : Clock
  Clock3 : Clock
  Constant2 : Constant  Value=0
  Constant3 : Constant
  Logical Operator2 : Logic  Operator=NOT  AllPortsSameDT=off
  Monostable1 : powerlib_extras/Control  Blocks/Monostable  EdgeDetect=Rising  t_mono=1000000  ic=0
  Switch2 : Switch  Threshold=0.15
  Switch3 : Switch  Threshold=0.15
  Trip : Outport
  wires:
  Clock2/1 -> Switch2/2
  Constant2/1 -> Switch2/3
  Constant3/1 -> Switch3/3
  Clock3/1 -> Switch3/2
  Switch2/1 -> Monostable1/1
  Monostable1/1 -> Logical Operator2/1
  Logical Operator2/1 -> Switch3/1
  Cond/1 -> Switch2/1
  Switch3/1 -> Trip/1

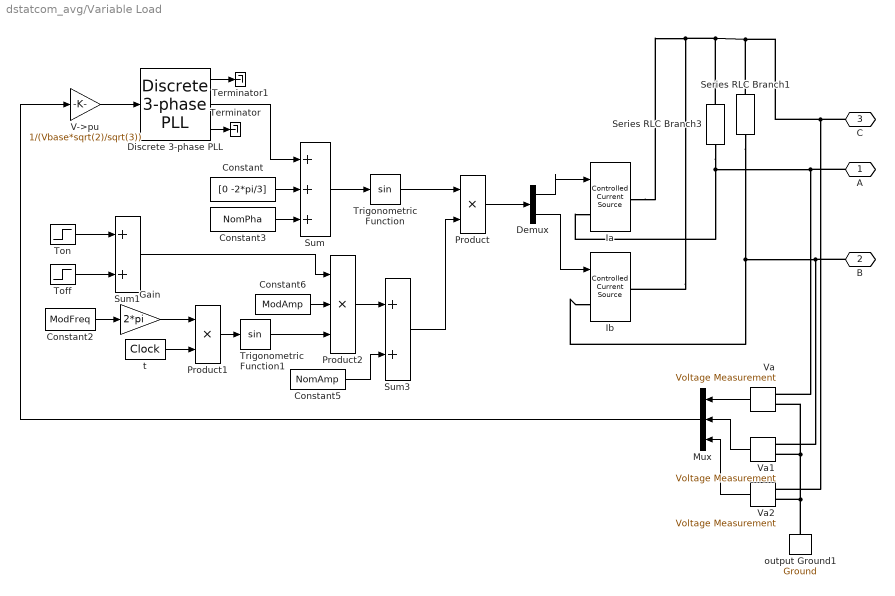
== system dstatcom_avg/Variable Load ==
  Constant : Constant  Value=[0 -2*pi/3]
  Constant2 : Constant  Value=ModFreq
  Constant3 : Constant  Value=NomPha
  Constant5 : Constant  Value=NomAmp
  Constant6 : Constant  Value=ModAmp
  Demux : Demux  Outputs=2
  Discrete 3-phase PLL : powerlib_extras/Discrete  Control Blocks/Discrete 3-phase PLL  Fmin=45  Par_Init=[0 60]  ParK=[60 1400]  Ts=Ts  AGC=off
  Gain : Gain  Gain=2*pi  SaturateOnIntegerOverflow=on  OutDataTypeStr=Inherit: Same as input  ParamDataTypeStr=Inherit: Same as input
  Ia : powerlib/Electrical Sources/Controlled Current Source  Description=source block  Initialize=on  Source_Type=AC  Amplitude=0  Phase=0  Frequency=0  Measurements=None
      settings: AttributesFormatString=\n
  Ib : powerlib/Electrical Sources/Controlled Current Source  Description=source block  Initialize=on  Source_Type=AC  Amplitude=0  Phase=0  Frequency=0  Measurements=None
      settings: AttributesFormatString=\n
  Mux : Mux  Inputs=3
  Product : Product  SaturateOnIntegerOverflow=on  InputSameDT=on  OutDataTypeStr=Inherit: Same as first input
  Product1 : Product  SaturateOnIntegerOverflow=on  InputSameDT=on  OutDataTypeStr=Inherit: Same as first input
  Product2 : Product  Inputs=3  SaturateOnIntegerOverflow=on  InputSameDT=on  OutDataTypeStr=Inherit: Same as first input
  Series RLC Branch1 : powerlib/Elements/Series RLC Branch  LConnTagsString=__new0  RConnTagsString=__new0  BranchType=R  Resistance=1e6  Inductance=1.0  SetiL0=off  InitialCurrent=0  Capacitance=1.0  Setx0=off  InitialVoltage=0  Measurements=None
  Series RLC Branch3 : powerlib/Elements/Series RLC Branch  LConnTagsString=__new0  RConnTagsString=__new0  BranchType=R  Resistance=1e6  Inductance=1.0  SetiL0=off  InitialCurrent=0  Capacitance=1.0  Setx0=off  InitialVoltage=0  Measurements=None
  Sum : Sum  Inputs=+++  SaturateOnIntegerOverflow=on  InputSameDT=on  OutDataTypeStr=Inherit: Same as first input
  Sum1 : Sum  SaturateOnIntegerOverflow=on  InputSameDT=on  OutDataTypeStr=Inherit: Same as first input
  Sum3 : Sum  SaturateOnIntegerOverflow=on  InputSameDT=on  OutDataTypeStr=Inherit: Same as first input
  Terminator : Terminator
  Terminator1 : Terminator
  Toff : Step  Time=Toff  After=-1  SampleTime=Ts
  Ton : Step  Time=Ton  SampleTime=Ts
  Trigonometric Function : Trigonometry
  Trigonometric Function1 : Trigonometry
  V->pu : Gain  Gain=1/(Vbase*sqrt(2)/sqrt(3))  SaturateOnIntegerOverflow=on  OutDataTypeStr=Inherit: Same as input  ParamDataTypeStr=Inherit: Same as input
  Va : powerlib/Measurements/Voltage Measurement  Tag=PoWeRsYsTeMmEaSuReMeNt  PhasorSimulation=off  OutputType=Magnitude  PSBequivalent=0
  Va1 : powerlib/Measurements/Voltage Measurement  Tag=PoWeRsYsTeMmEaSuReMeNt  PhasorSimulation=off  OutputType=Magnitude  PSBequivalent=0
  Va2 : powerlib/Measurements/Voltage Measurement  Tag=PoWeRsYsTeMmEaSuReMeNt  PhasorSimulation=off  OutputType=Magnitude  PSBequivalent=0
  output Ground1 : powerlib/Elements/Ground  LConnTagsString=a  RConnTagsString=__newr0
  t : DigitalClock  SampleTime=Ts
  A : PMIOPort  Port=1  Side=Left
  B : PMIOPort  Port=2  Side=Left
  C : PMIOPort  Port=3  Side=Left
  wires:
  Sum1/1 -> Product2/1
  Toff/1 -> Sum1/2
  Ton/1 -> Sum1/1
  Constant6/1 -> Product2/2
  Trigonometric Function1/1 -> Product2/3
  Constant5/1 -> Sum3/2
  Product2/1 -> Sum3/1
  Sum3/1 -> Product/2
  Product1/1 -> Trigonometric Function1/1
  t/1 -> Product1/2
  Gain/1 -> Product1/1
  Constant2/1 -> Gain/1
  Constant3/1 -> Sum/3
  Mux/1 -> V->pu/1
  Discrete 3-phase PLL/2 -> Sum/1
  V->pu/1 -> Discrete 3-phase PLL/1
  Discrete 3-phase PLL/3 -> Terminator/1
  Discrete 3-phase PLL/1 -> Terminator1/1
  Product/1 -> Demux/1
  Trigonometric Function/1 -> Product/1
  Sum/1 -> Trigonometric Function/1
  Constant/1 -> Sum/2
  Va2/1 -> Mux/3
  Va1/1 -> Mux/2
  Va/1 -> Mux/1
  Demux/2 -> Ib/1
  Demux/1 -> Ia/1
  connections:
  output Ground1/LConn1 -- Va2/LConn2 -- Va1/LConn2 -- Va/LConn2
  Ib/LConn1 -- Series RLC Branch1/LConn1 -- B/RConn1 -- Va1/LConn1
  Ia/LConn1 -- Series RLC Branch3/LConn1 -- A/RConn1 -- Va/LConn1
  Series RLC Branch1/RConn1 -- Series RLC Branch3/RConn1 -- Ia/RConn1 -- Ib/RConn1 -- C/RConn1 -- Va2/LConn1

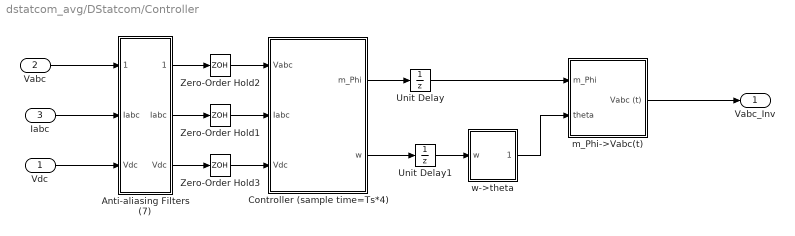
== system dstatcom_avg/DStatcom/Controller ==
  Vdc : Inport  PortDimensions=1
  Vabc : Inport  Port=2  PortDimensions=3
  Iabc : Inport  Port=3  PortDimensions=3
  Anti-aliasing Filters (7) : Subsystem  mask(Anti-aliasing (2nd order lowpass)){Fc=2000, Ts=Ts}
      mask prompts: Fc "Cut-off frequency (Hz):"; Ts "Sample time:"
  Controller (sample time=Ts*4) : Subsystem
  Unit Delay : UnitDelay  SampleTime=Ts*4
  Unit Delay1 : UnitDelay  SampleTime=Ts*4
  Zero-Order Hold1 : ZeroOrderHold  SampleTime=Ts*4
  Zero-Order Hold2 : ZeroOrderHold  SampleTime=Ts*4
  Zero-Order Hold3 : ZeroOrderHold  SampleTime=Ts*4
  m_Phi->Vabc(t) : Subsystem
  w->theta : Subsystem
  Vabc_Inv : Outport
  wires:
  w->theta/1(theta) -> m_Phi->Vabc(t)/2(theta)
  Unit Delay1/1 -> w->theta/1(w)
  Controller (sample time=Ts*4)/2(w) -> Unit Delay1/1
  m_Phi->Vabc(t)/1(Vabc (t)) -> Vabc_Inv/1
  Unit Delay/1 -> m_Phi->Vabc(t)/1(m_Phi)
  Controller (sample time=Ts*4)/1(m_Phi) -> Unit Delay/1
  Zero-Order Hold3/1 -> Controller (sample time=Ts*4)/3(Vdc)
  Zero-Order Hold1/1 -> Controller (sample time=Ts*4)/2(Iabc)
  Zero-Order Hold2/1 -> Controller (sample time=Ts*4)/1(Vabc)
  Vdc/1 -> Anti-aliasing Filters (7)/3("Vdc ")
  Iabc/1 -> Anti-aliasing Filters (7)/2("Iabc ")
  Vabc/1 -> Anti-aliasing Filters (7)/1(Vabc)
  Anti-aliasing Filters (7)/3(" Vdc") -> Zero-Order Hold3/1
  Anti-aliasing Filters (7)/2(Iabc) -> Zero-Order Hold1/1
  Anti-aliasing Filters (7)/1(" Vabc") -> Zero-Order Hold2/1

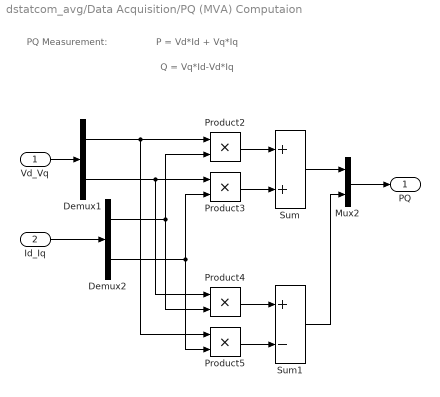
== system dstatcom_avg/Data Acquisition/PQ (MVA) Computaion ==
  note: PQ Measurement:
  note: Q = Vq*Id-Vd*Iq
  note: P = Vd*Id + Vq*Iq
  Vd_Vq : Inport  PortDimensions=2
  Id_Iq : Inport  Port=2  PortDimensions=2
  Demux1 : Demux  Outputs=2
  Demux2 : Demux  Outputs=2
  Mux2 : Mux  Inputs=2
  Product{2..5} (4 alike) : Product  SaturateOnIntegerOverflow=on  InputSameDT=on  OutDataTypeStr=Inherit: Same as first input
  Sum : Sum  SaturateOnIntegerOverflow=on  InputSameDT=on  OutDataTypeStr=Inherit: Same as first input
  Sum1 : Sum  Inputs=+-  SaturateOnIntegerOverflow=on  InputSameDT=on  OutDataTypeStr=Inherit: Same as first input
  PQ : Outport
  wires:
  Demux2/2 -> Product5/2, Product3/2
  Demux1/1 -> Product5/1, Product2/1
  Demux2/1 -> Product4/2, Product2/2
  Demux1/2 -> Product4/1, Product3/1
  Id_Iq/1 -> Demux2/1
  Vd_Vq/1 -> Demux1/1
  Sum1/1 -> Mux2/2
  Sum/1 -> Mux2/1
  Product5/1 -> Sum1/2
  Product4/1 -> Sum1/1
  Product3/1 -> Sum/2
  Product2/1 -> Sum/1
  Mux2/1 -> PQ/1

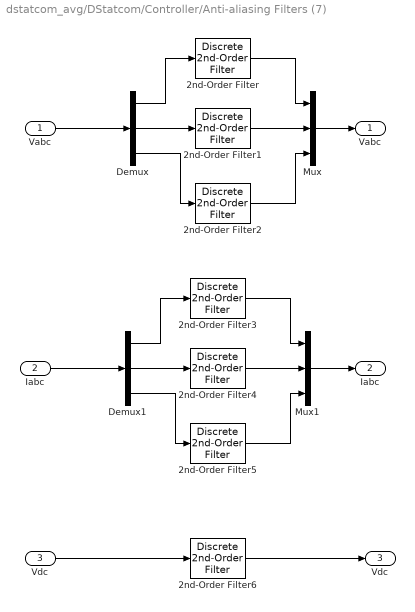
== system dstatcom_avg/DStatcom/Controller/Anti-aliasing Filters (7) ==
  Vabc : Inport  PortDimensions=3
  "Iabc " : Inport  Port=2  PortDimensions=3
  "Vdc " : Inport  Port=3  PortDimensions=1
  2nd-Order Filter{,1..6} (7 alike) : powerlib_extras/Discrete  Control Blocks/Discrete  2nd-Order Filter  FilterType=Lowpass  Fo=Fc  Zeta=0.707  Ts=Ts  Initialize=off  Vac_Init=[0.8 -25 60]  Vdc_Init=-0.4  PlotResponse=off  param1=[1 5000 0.1]
  Demux : Demux  Outputs=3
  Demux1 : Demux  Outputs=3
  Mux : Mux  Inputs=3
  Mux1 : Mux  Inputs=3
  " Vabc" : Outport
  Iabc : Outport  Port=2
  " Vdc" : Outport  Port=3
  wires:
  "Iabc "/1 -> Demux1/1
  Demux1/2 -> 2nd-Order Filter4/1
  Demux1/3 -> 2nd-Order Filter5/1
  2nd-Order Filter5/1 -> Mux1/3
  2nd-Order Filter4/1 -> Mux1/2
  Mux1/1 -> Iabc/1
  2nd-Order Filter3/1 -> Mux1/1
  Demux1/1 -> 2nd-Order Filter3/1
  Demux/2 -> 2nd-Order Filter1/1
  Demux/3 -> 2nd-Order Filter2/1
  2nd-Order Filter2/1 -> Mux/3
  2nd-Order Filter1/1 -> Mux/2
  2nd-Order Filter6/1 -> " Vdc"/1
  "Vdc "/1 -> 2nd-Order Filter6/1
  Mux/1 -> " Vabc"/1
  2nd-Order Filter/1 -> Mux/1
  Vabc/1 -> Demux/1
  Demux/1 -> 2nd-Order Filter/1
